simulink model "compare_pids_ind"  (R2020b)
settings: Solver=VariableStepAuto  StartTime=0.0  StopTime=150  RelTol=1e-3
values from neighbouring files (symbols this model uses):
  kp_cc_strejc = (1.35 / alpha_cc_strejc )*(1 + ((0.18 * tau_cc_strejc)/ (1 - tau_cc_strejc)))    [sem1.m]
  kp_cc_strejc_ind = (kp_cc_strejc/2) * (1+sqrt(1-4*td_cc_strejc/ti_cc_strejc))    [sem1.m]
  plant_1 = tf([K], conv([T1,1],[T2,1]))    [plant.m]
  td_cc_strejc = ((0.37 - 0.37* tau_cc_strejc)/(1 - 0.81 * tau_cc_strejc)) * l_cc_strejc    [sem1.m]
  td_cc_strejc_ind = (td_cc_strejc/2) * (1+sqrt(1-4*td_cc_strejc/ti_cc_strejc))    [sem1.m]
  ti_cc_strejc = ((2.50 - 2.0 * tau_cc_strejc)/(1 - 0.39 * tau_cc_strejc)) * l_cc_strejc    [sem1.m]
  ti_cc_strejc_ind = (ti_cc_strejc/2) * (1+sqrt(1-4*td_cc_strejc/ti_cc_strejc))    [sem1.m]
settings Model: Creator=rafael  LastModifiedBy=rafael

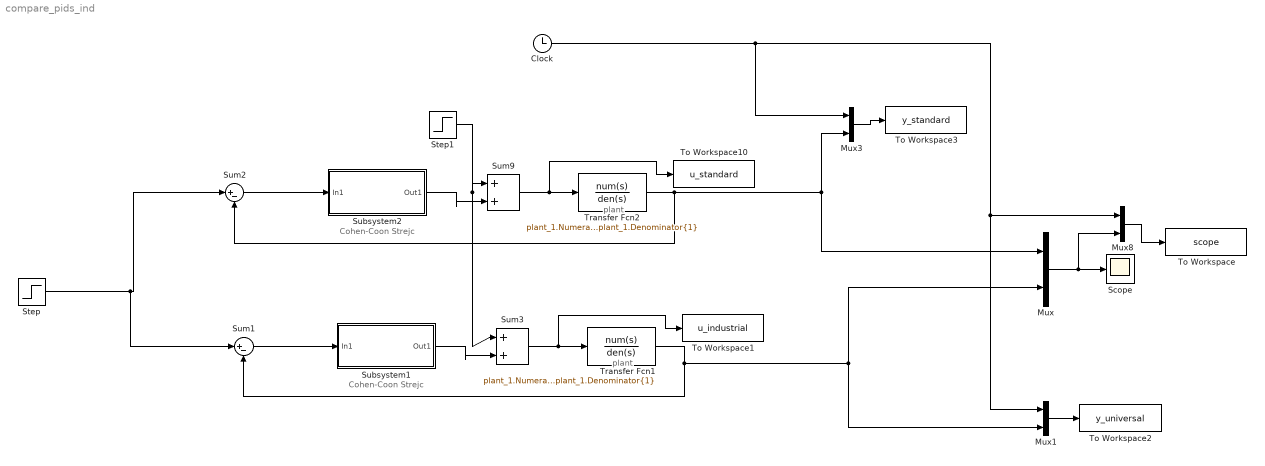
== system compare_pids_ind ==
  note: Cohen-Coon Strejc
  note: plant
  note: Cohen-Coon Strejc
  note: plant
  Clock : Clock
  Mux{,1,3,8} (4 alike) : Mux  Inputs=2
  Scope : Scope
  Step : Step  Time=0  SampleTime=0
  Step1 : Step  Time=80  After=-0.5  SampleTime=0
  Subsystem1 : Subsystem  mask{kp=kp_cc_strejc_ind, ti=ti_cc_strejc_ind, td=td_cc_strejc_ind}
      mask prompts: kp "Proportional gain (kp)"; ti "Integral time (ti)"; td "Derrivative_time (td)"
      mask help: u(s)=kp*(1 + (1/ti)/s + td*s)
      mask Help: /*No help for now*/
      mask Display: disp(' industrialPID '), port_label('input',1,'e'), port_label('output',1,'u')
  Subsystem2 : Subsystem  mask{kp=kp_cc_strejc, ti=ti_cc_strejc, td=td_cc_strejc}
      mask prompts: kp "Proportional gain (kp)"; ti "Integral time (ti)"; td "Derrivative_time (td)"
      mask help: u(s)=kp*(1 + (1/ti)/s + td*s)
      mask Help: /*No help for now*/
      mask Display: disp(' standardPID '), port_label('input',1,'e'), port_label('output',1,'u')
  Sum1 : Sum  Inputs=|+-
  Sum2 : Sum  Inputs=|+-
  Sum3 : Sum  Inputs=|++
  Sum9 : Sum  Inputs=|++
  To Workspace : ToWorkspace  VariableName=scope  SaveFormat=Timeseries  SampleTime=-1
  To Workspace1 : ToWorkspace  VariableName=u_industrial  SampleTime=-1
      settings: Save2DSignal=2-D array (concatenate along first dimension)
  To Workspace10 : ToWorkspace  VariableName=u_standard  SampleTime=-1
      settings: Save2DSignal=2-D array (concatenate along first dimension)
  To Workspace2 : ToWorkspace  VariableName=y_universal  SampleTime=-1
      settings: Save2DSignal=2-D array (concatenate along first dimension)
  To Workspace3 : ToWorkspace  VariableName=y_standard  SampleTime=-1
      settings: Save2DSignal=2-D array (concatenate along first dimension)
  Transfer Fcn1 : TransferFcn  Numerator=plant_1.Numerator{1}  Denominator=plant_1.Denominator{1}
  Transfer Fcn2 : TransferFcn  Numerator=plant_1.Numerator{1}  Denominator=plant_1.Denominator{1}
  wires:
  Mux/1 -> Mux8/2, Scope/1
  Sum2/1 -> Subsystem2/1(In1)
  Transfer Fcn2/1 -> Sum2/2, Mux3/2, Mux/1
  Mux3/1 -> To Workspace3/1
  Clock/1 -> Mux3/1, Mux8/1, Mux1/1
  Mux8/1 -> To Workspace/1
  Sum9/1 -> To Workspace10/1, Transfer Fcn2/1
  Subsystem2/1(Out1) -> Sum9/2
  Subsystem1/1(Out1) -> Sum3/2
  Sum1/1 -> Subsystem1/1(In1)
  Step/1 -> Sum1/1, Sum2/1
  Sum3/1 -> To Workspace1/1, Transfer Fcn1/1
  Mux1/1 -> To Workspace2/1
  Transfer Fcn1/1 -> Mux/2, Mux1/2, Sum1/2
  Step1/1 -> Sum3/1, Sum9/1

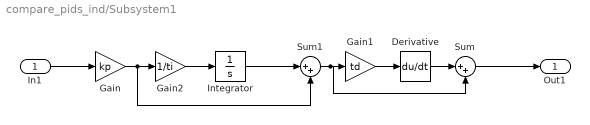
== system compare_pids_ind/Subsystem1 ==
  In1 : Inport
  Derivative : Derivative
  Gain : Gain  Gain=kp
  Gain1 : Gain  Gain=td
  Gain2 : Gain  Gain=1/ti
  Integrator : Integrator
  Sum : Sum  Inputs=|++
  Sum1 : Sum  Inputs=|++
  Out1 : Outport
  wires:
  Gain1/1 -> Derivative/1
  Gain/1 -> Sum1/2, Gain2/1
  In1/1 -> Gain/1
  Gain2/1 -> Integrator/1
  Integrator/1 -> Sum1/1
  Sum1/1 -> Sum/2, Gain1/1
  Derivative/1 -> Sum/1
  Sum/1 -> Out1/1

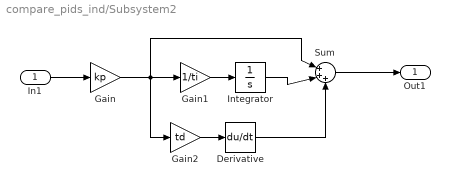
== system compare_pids_ind/Subsystem2 ==
  In1 : Inport
  Derivative : Derivative
  Gain : Gain  Gain=kp
  Gain1 : Gain  Gain=1/ti
  Gain2 : Gain  Gain=td
  Integrator : Integrator
  Sum : Sum  Inputs=|+++
  Out1 : Outport
  wires:
  Sum/1 -> Out1/1
  In1/1 -> Gain/1
  Derivative/1 -> Sum/3
  Gain/1 -> Gain2/1, Gain1/1, Sum/1
  Gain2/1 -> Derivative/1
  Integrator/1 -> Sum/2
  Gain1/1 -> Integrator/1
